simulink model "labpinv2"  (Simulink 6.3)
settings: Solver=ode1  SolverMode=SingleTasking  StartTime=0.0  StopTime=inf  FixedStep=0.001  RelTol=1e-3
values from neighbouring files (symbols this model uses):
  K = [0,0,0,0,0]    [setup_lab_ip01_2_sip.m]
  wcf = 2 * pi * 10    (= 62.8318530718)    [setup_lab_ip01_2_sip.m]
  X_LIM_ENABLE = 1    [setup_lab_ip01_2_sip.m]
  X_MAX = 0.35    [setup_lab_ip01_2_sip.m]
  X_MIN = - X_MAX    (= -0.35)    [setup_lab_ip01_2_sip.m]
  zetaf = 0.9    [setup_lab_ip01_2_sip.m]
libraries: qctools x5, simulink x2
settings Model: LastModifiedBy=localadmin  ExtModeArmWhenConnect=off  BufferReuse=off  StrictBusMsg=None
settings ConfigSet: SimulationMode=external
settings OptimizationCC: BooleanDataType=off  InlineInvariantSignals=on  OptimizeBlockIOStorage=off  BufferReuse=off  ExpressionFolding=off  LocalBlockOutputs=off
settings RTWCC: SystemTargetFile=wincon.tlc  MakeCommand=make_wc  TemplateMakefile=wc_default_tmf  Description=WinCon Target  ProcessScript=wincon_make_rtw_hook
settings STFCustomTargetCC: TargetFcnLib=ansi_tfl_tmw.mat  GenFloatMathFcnCalls=ANSI_C  ModelReferenceCompliant=off  SystemTargetFile=wincon.tlc
settings GRTTargetCC: ModelReferenceCompliant=off  MatFileLogging=off  ExtMode=on  ExtModeTransport=2  ExtModeMexFile=wc_comm
settings CustomProperty: Value=on

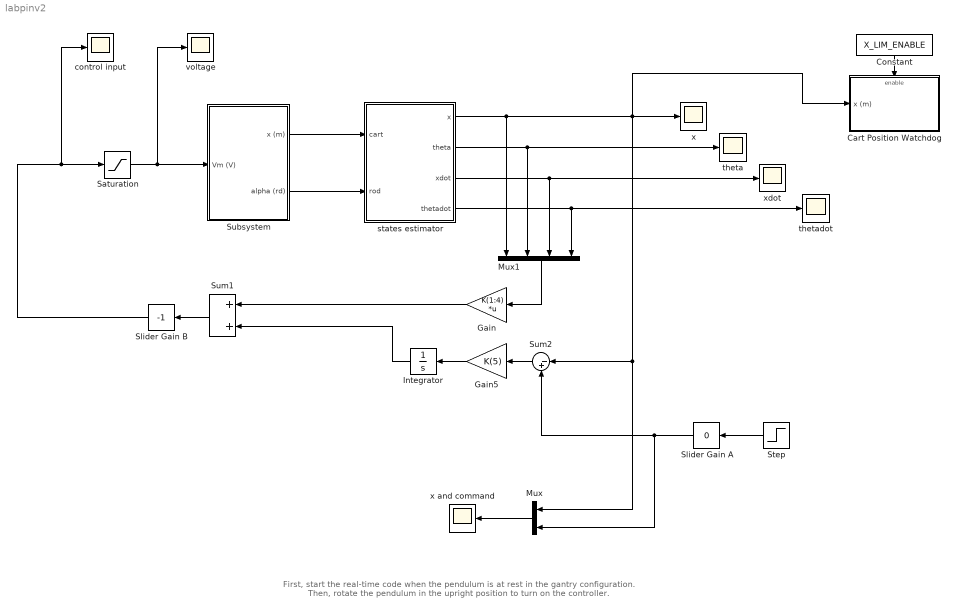
== system labpinv2 ==
  note: First, start the real-time code when the pendulum is at rest in the gantry configuration.
      | Then, rotate the pendulum in the upright position to turn on the controller.
  Cart Position Watchdog : Subsystem  TreatAsAtomicUnit=on
  Constant : Constant  Orientation=down  Value=X_LIM_ENABLE
  Gain : Gain  Orientation=left  Gain=K(1:4)  Multiplication=Matrix(K*u)
  Gain5 : Gain  Orientation=left  Gain=K(5)
  Integrator : Integrator  Orientation=left
  Mux : Mux  Orientation=left  Inputs=2
  Mux1 : Mux  Orientation=down
  Saturation : Saturate  UpperLimit=6  LowerLimit=-6
  Slider Gain A : simulink/Math Operations/Slider Gain  Orientation=left  low=-0.2  gain=0  high=0.2
  Slider Gain B : simulink/Math Operations/Slider Gain  Orientation=left  low=-1  gain=-1  high=1
  Step : Step  Orientation=left  Time=0  SampleTime=0
  Subsystem : Subsystem
  Sum1 : Sum  Orientation=left
  Sum2 : Sum  Orientation=left  Inputs=|-+
  control input : Scope
      settings: SaveName=ScopeData3
  states estimator : Subsystem
  theta : Scope
  thetadot : Scope
      settings: SaveName=ScopeData2
  voltage : Scope
      settings: SaveName=ScopeData5
  x : Scope
      settings: SaveName=ScopeData4
  x and command : Scope
      settings: SaveName=ScopeData6
  xdot : Scope
  wires:
  Slider Gain B/1 -> Saturation/1, control input/1
  states estimator/1(x) -> Cart Position Watchdog/1(x (m)), Mux1/1, x/1, Sum2/1, Mux/1
  states estimator/2(theta) -> theta/1, Mux1/2
  states estimator/3(xdot) -> xdot/1, Mux1/3
  states estimator/4(thetadot) -> thetadot/1, Mux1/4
  Sum1/1 -> Slider Gain B/1
  Saturation/1 -> voltage/1, Subsystem/1(Vm (V))
  Sum2/1 -> Gain5/1
  Gain5/1 -> Integrator/1
  Slider Gain A/1 -> Sum2/2, Mux/2
  Step/1 -> Slider Gain A/1
  Constant/1 -> Cart Position Watchdog/Enable
  Mux/1 -> x and command/1
  Subsystem/1(x (m)) -> states estimator/1(cart)
  Subsystem/2(alpha (rd)) -> states estimator/2(rod)
  Mux1/1 -> Gain/1
  Integrator/1 -> Sum1/2
  Gain/1 -> Sum1/1

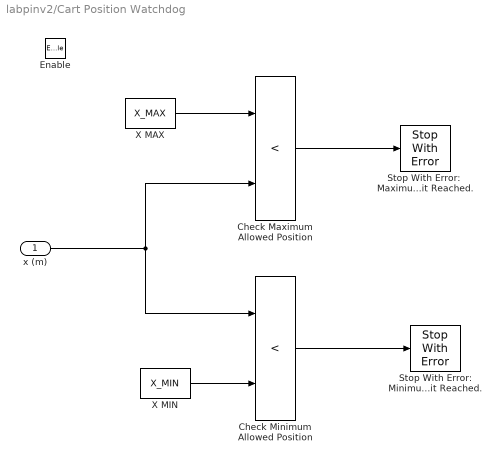
== system labpinv2/Cart Position Watchdog ==
  x (m) : Inport
  Enable : EnablePort
  Check Maximum Allowed Position : RelationalOperator  Operator=<  ZeroCross=off  InputSameDT=on
  Check Minimum Allowed Position : RelationalOperator  Operator=<  ZeroCross=off  InputSameDT=on
  Stop With Error: Minimum Limit Reached. : qctools/Extra Sinks/Stop With Error  errMsg=Minimum Position Limit reached.
  Stop With Error:  Maximum Limit Reached. : qctools/Extra Sinks/Stop With Error  errMsg=Maximum Position Limit reached.
  X MAX : Constant  Value=X_MAX
  X MIN : Constant  Value=X_MIN
  wires:
  Check Maximum Allowed Position/1 -> Stop With Error:  Maximum Limit Reached./1
  x (m)/1 -> Check Minimum Allowed Position/1, Check Maximum Allowed Position/2
  X MIN/1 -> Check Minimum Allowed Position/2
  Check Minimum Allowed Position/1 -> Stop With Error: Minimum Limit Reached./1
  X MAX/1 -> Check Maximum Allowed Position/1

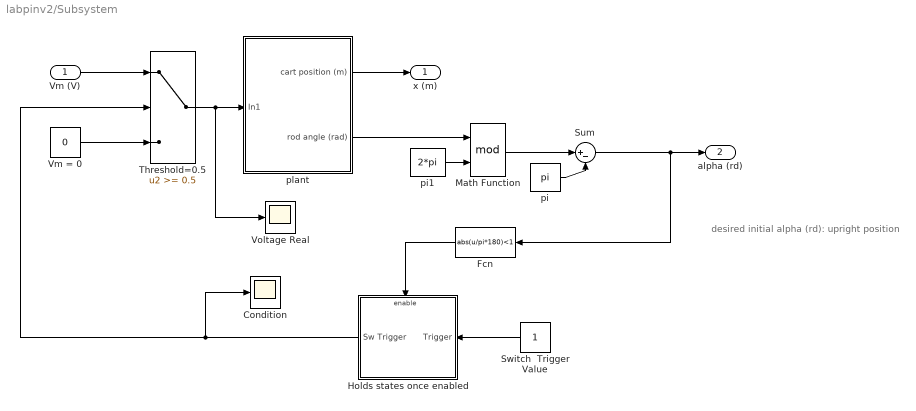
== system labpinv2/Subsystem ==
  note: desired initial alpha (rd):
      | upright position
  Vm (V) : Inport
  Condition : Scope
      settings: SaveName=ScopeData7
  Fcn : Fcn  Orientation=left  Expr=abs(u/pi*180)<1
  Holds states once enabled : Subsystem  Orientation=left  TreatAsAtomicUnit=on
  Math Function : Math  Operator=mod  SaturateOnIntegerOverflow=on
  Sum : Sum  Inputs=|+-  SaturateOnIntegerOverflow=on  InputSameDT=on
  Switch  Trigger Value : Constant  Orientation=left
  Threshold=0.5 : Switch  Threshold=0.5  SaturateOnIntegerOverflow=on  InputSameDT=on
  Vm = 0 : Constant  Value=0
  Voltage Real : Scope
      settings: SaveName=ScopeData8
  pi : Constant  Value=pi
  pi1 : Constant  Value=2*pi
  plant : Subsystem
  x (m) : Outport  InitialOutput=0
  alpha (rd) : Outport  Port=2  InitialOutput=0
  wires:
  plant/1(cart position (m)) -> x (m)/1
  plant/2(rod angle (rad)) -> Math Function/1
  pi1/1 -> Math Function/2
  Switch  Trigger Value/1 -> Holds states once enabled/1(Trigger)
  Threshold=0.5/1 -> plant/1(In1), Voltage Real/1
  Vm (V)/1 -> Threshold=0.5/1
  Vm = 0/1 -> Threshold=0.5/3
  pi/1 -> Sum/2
  Sum/1 -> alpha (rd)/1, Fcn/1
  Math Function/1 -> Sum/1
  Fcn/1 -> Holds states once enabled/Enable
  Holds states once enabled/1(Sw Trigger) -> Threshold=0.5/2, Condition/1

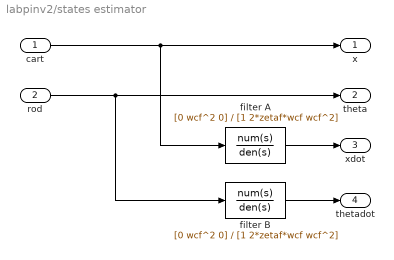
== system labpinv2/states estimator ==
  cart : Inport
  rod : Inport  Port=2
  filter A : TransferFcn  Numerator=[0 wcf^2 0]  Denominator=[1 2*zetaf*wcf wcf^2]
  filter B : TransferFcn  Numerator=[0 wcf^2 0]  Denominator=[1 2*zetaf*wcf wcf^2]
  x : Outport
  theta : Outport  Port=2
  xdot : Outport  Port=3
  thetadot : Outport  Port=4
  wires:
  cart/1 -> x/1, filter A/1
  rod/1 -> theta/1, filter B/1
  filter A/1 -> xdot/1
  filter B/1 -> thetadot/1

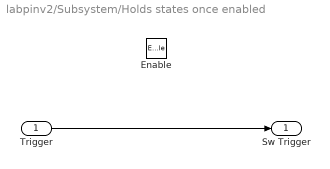
== system labpinv2/Subsystem/Holds states once enabled ==
  Trigger : Inport
  Enable : EnablePort
  Sw Trigger : Outport  InitialOutput=[0]
  wires:
  Trigger/1 -> Sw Trigger/1

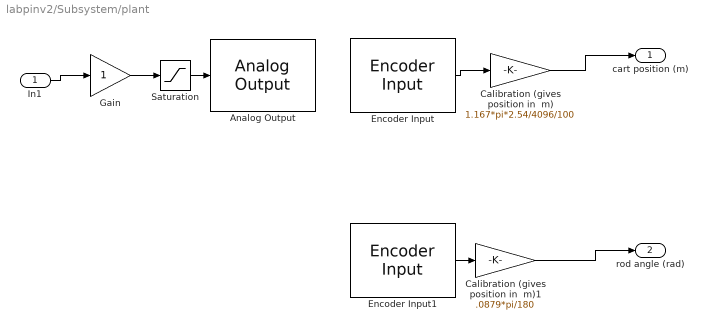
== system labpinv2/Subsystem/plant ==
  In1 : Inport
  Analog Output : qctools/Quanser Q4 Series/Analog Output  boardNumber=0  channels=0  modesVect=0  rangesVect=10  initialVect=0  finalVect=0  sampleTime=-1  inputVolts=on  simulationOutput=off
  Calibration (gives position in  m) : Gain  Gain=1.167*pi*2.54/4096/100  SaturateOnIntegerOverflow=on
  Calibration (gives position in  m)1 : Gain  Gain=.0879*pi/180  SaturateOnIntegerOverflow=on
  Encoder Input : qctools/Quanser Q4 Series/Encoder Input  boardNumber=0  channels=0  initial=0  preserveCounts=off  sampleTime=default_sample_time  quadratureStr=4X  modeStr=Normal  flagString=FLG1 is IDX and FLG2 is E  prescale=1  frequency=16666666.6667  use33MHzClock=off  bcd=off  enableIndex=on  synchronousIndex=on  indexPolarity=on  reloadOnIndex=off  simulationInput=off
  Encoder Input1 : qctools/Quanser Q4 Series/Encoder Input  boardNumber=0  channels=1  initial=0  preserveCounts=off  sampleTime=default_sample_time  quadratureStr=4X  modeStr=Normal  flagString=FLG1 is IDX and FLG2 is E  prescale=1  frequency=16666666.6667  use33MHzClock=off  bcd=off  enableIndex=on  synchronousIndex=on  indexPolarity=on  reloadOnIndex=off  simulationInput=off
  Gain : Gain  SaturateOnIntegerOverflow=on
  Saturation : Saturate  UpperLimit=6  LowerLimit=-6
  cart position (m) : Outport
  rod angle (rad) : Outport  Port=2
  wires:
  Encoder Input/1 -> Calibration (gives position in  m)/1
  Calibration (gives position in  m)/1 -> cart position (m)/1
  Calibration (gives position in  m)1/1 -> rod angle (rad)/1
  Encoder Input1/1 -> Calibration (gives position in  m)1/1
  Saturation/1 -> Analog Output/1
  In1/1 -> Gain/1
  Gain/1 -> Saturation/1
